simulink model "model_SCARA_PD"  (R2022b)
settings: Solver=VariableStepAuto  StartTime=0.0  StopTime=times_way(end)  RelTol=1e-3
undefined symbols (not defined in the file or in its folder): dt_animation, phi_0, psi_0, q1_0, q1_dot_0, q2_0, q2_dot_0, q3_0, q3_dot_0, q4_0, q4_dot_0, theta_0, x_0, y_0, z_0
libraries: robotcorelib x1
settings Model: Creator=anton  LastModifiedBy=angel

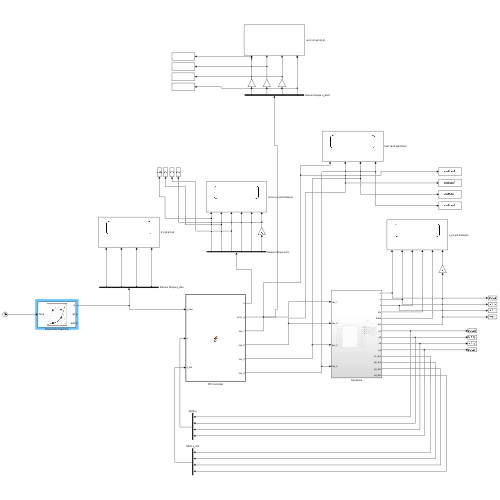
[thumbnail: Simulink's stored preview of the top-level diagram]
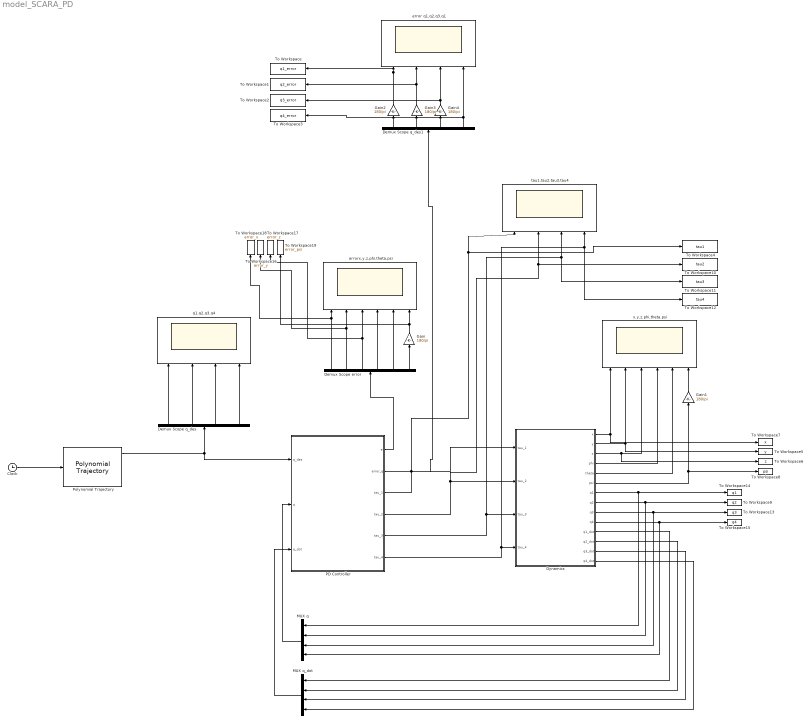
== system model_SCARA_PD ==
  Clock : Clock
  Demux Scope error : Demux  Outputs=6
  Demux Scope q_des : Demux
  Demux Scope q_des1 : Demux
  Dynamics : Subsystem
  Gain{,1..4} (5 alike) : Gain  Gain=180/pi
  MUX q : Mux
  MUX q_dot : Mux
  PD Controller : MATLAB Function  TreatAsAtomicUnit=on
  Polynomial Trajectory : robotcorelib/Polynomial Trajectory  WaypointSource=Internal  Waypoints=waypoints  TimePoints=times_way  TimeInterval=[ 1, 4 ]  Method=Cubic Polynomial  ParameterSource=Internal  VelocityBoundaryCondition=vel_boundary_condit  AccelerationBoundaryCondition=zeros( 2, 5 )  SimulateUsing=Interpreted execution
  To Workspace : ToWorkspace  VariableName=q1_error  SampleTime=dt_animation
  To Workspace1 : ToWorkspace  VariableName=q2_error  SampleTime=dt_animation
  To Workspace10 : ToWorkspace  VariableName=tau2  SampleTime=dt_animation
  To Workspace11 : ToWorkspace  VariableName=tau3  SampleTime=dt_animation
  To Workspace12 : ToWorkspace  VariableName=tau4  SampleTime=dt_animation
  To Workspace13 : ToWorkspace  VariableName=q3  SampleTime=dt_animation
  To Workspace14 : ToWorkspace  VariableName=q1  SampleTime=dt_animation
  To Workspace15 : ToWorkspace  VariableName=q4  SampleTime=dt_animation
  To Workspace16 : ToWorkspace  VariableName=error_y  SampleTime=dt_animation
  To Workspace17 : ToWorkspace  VariableName=error_z  SampleTime=dt_animation
  To Workspace18 : ToWorkspace  VariableName=error_x  SampleTime=dt_animation
  To Workspace19 : ToWorkspace  VariableName=error_psi  SampleTime=dt_animation
  To Workspace2 : ToWorkspace  VariableName=q3_error  SampleTime=dt_animation
  To Workspace3 : ToWorkspace  VariableName=q4_error  SampleTime=dt_animation
  To Workspace4 : ToWorkspace  VariableName=tau1  SampleTime=dt_animation
  To Workspace5 : ToWorkspace  VariableName=y  SampleTime=dt_animation
  To Workspace6 : ToWorkspace  VariableName=z  SampleTime=dt_animation
  To Workspace7 : ToWorkspace  VariableName=x  SampleTime=dt_animation
  To Workspace8 : ToWorkspace  VariableName=psi  SampleTime=dt_animation
  To Workspace9 : ToWorkspace  VariableName=q2  SampleTime=dt_animation
  error q1,q2,q3,q1 : Scope  NumInputPorts=4
  errorx,y,z,phi,theta,psi : Scope  NumInputPorts=6
  q1,q2,q3,q4 : Scope  NumInputPorts=4
  tau1,tau2,tau3,tau4 : Scope  NumInputPorts=4
  x,y,z,phi,theta,psi : Scope  NumInputPorts=6
  wires:
  Dynamics/7(q1) -> To Workspace14/1, MUX q/1
  Dynamics/8(q2) -> To Workspace9/1, MUX q/2
  Dynamics/9(q3) -> To Workspace13/1, MUX q/3
  Dynamics/10(q4) -> To Workspace15/1, MUX q/4
  Dynamics/11(q1_dot) -> MUX q_dot/1
  Dynamics/12(q2_dot) -> MUX q_dot/2
  Dynamics/13(q3_dot) -> MUX q_dot/3
  Dynamics/14(q4_dot) -> MUX q_dot/4
  MUX q/1 -> PD Controller/2(q)
  MUX q_dot/1 -> PD Controller/3(q_dot)
  Clock/1 -> Polynomial Trajectory/1
  Polynomial Trajectory/1 -> Demux Scope q_des/1, PD Controller/1(q_des)
  Demux Scope q_des/1 -> q1,q2,q3,q4/1
  Demux Scope q_des/2 -> q1,q2,q3,q4/2
  Demux Scope q_des/3 -> q1,q2,q3,q4/3
  Demux Scope q_des/4 -> q1,q2,q3,q4/4
  Demux Scope error/4 -> errorx,y,z,phi,theta,psi/4
  Demux Scope error/3 -> To Workspace17/1, errorx,y,z,phi,theta,psi/3
  Demux Scope error/2 -> To Workspace16/1, errorx,y,z,phi,theta,psi/2
  Demux Scope error/1 -> To Workspace18/1, errorx,y,z,phi,theta,psi/1
  Demux Scope error/5 -> errorx,y,z,phi,theta,psi/5
  Demux Scope error/6 -> Gain/1
  PD Controller/1(e) -> Demux Scope error/1
  Dynamics/6(psi) -> To Workspace8/1, Gain1/1
  Dynamics/1(x) -> To Workspace7/1, x,y,z,phi,theta,psi/1
  Dynamics/2(y) -> To Workspace5/1, x,y,z,phi,theta,psi/2
  Dynamics/3(z) -> To Workspace6/1, x,y,z,phi,theta,psi/3
  Dynamics/4(phi) -> x,y,z,phi,theta,psi/4
  Dynamics/5(theta) -> x,y,z,phi,theta,psi/5
  Gain/1 -> To Workspace19/1, errorx,y,z,phi,theta,psi/6
  PD Controller/6(tau_4) -> tau1,tau2,tau3,tau4/4, To Workspace12/1, Dynamics/4(tau_4)
  PD Controller/5(tau_3) -> tau1,tau2,tau3,tau4/3, To Workspace11/1, Dynamics/3(tau_3)
  PD Controller/4(tau_2) -> tau1,tau2,tau3,tau4/2, To Workspace10/1, Dynamics/2(tau_2)
  PD Controller/3(tau_1) -> tau1,tau2,tau3,tau4/1, To Workspace4/1, Dynamics/1(tau_1)
  Gain1/1 -> x,y,z,phi,theta,psi/6
  PD Controller/2(error_q) -> Demux Scope q_des1/1
  Demux Scope q_des1/2 -> Gain3/1
  Demux Scope q_des1/1 -> Gain2/1
  Demux Scope q_des1/3 -> Gain4/1
  Demux Scope q_des1/4 -> To Workspace3/1, error q1,q2,q3,q1/4
  Gain2/1 -> To Workspace/1, error q1,q2,q3,q1/1
  Gain3/1 -> error q1,q2,q3,q1/2, To Workspace1/1
  Gain4/1 -> error q1,q2,q3,q1/3, To Workspace2/1

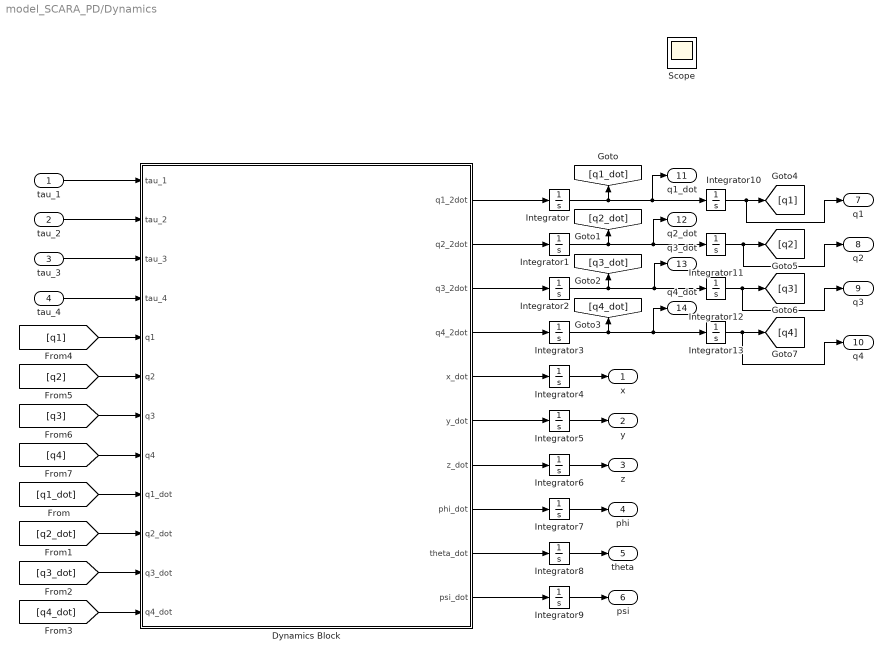
== system model_SCARA_PD/Dynamics ==
  tau_1 : Inport
  tau_2 : Inport  Port=2
  tau_3 : Inport  Port=3
  tau_4 : Inport  Port=4
  Dynamics Block : MATLAB Function  TreatAsAtomicUnit=on
  Integrator : Integrator  InitialCondition=q1_dot_0
  Integrator1 : Integrator  InitialCondition=q2_dot_0
  Integrator10 : Integrator  InitialCondition=q1_0  WrapState=on
  Integrator11 : Integrator  InitialCondition=q2_0  WrapState=on
  Integrator12 : Integrator  InitialCondition=q3_0  WrapState=on
  Integrator13 : Integrator  InitialCondition=q4_0
  Integrator2 : Integrator  InitialCondition=q3_dot_0
  Integrator3 : Integrator  InitialCondition=q4_dot_0
  Integrator4 : Integrator  InitialCondition=x_0
  Integrator5 : Integrator  InitialCondition=y_0
  Integrator6 : Integrator  InitialCondition=z_0
  Integrator7 : Integrator  InitialCondition=phi_0
  Integrator8 : Integrator  InitialCondition=theta_0
  Integrator9 : Integrator  InitialCondition=psi_0
  Scope : Scope  NumInputPorts=4
  x : Outport
  y : Outport  Port=2
  z : Outport  Port=3
  phi : Outport  Port=4
  theta : Outport  Port=5
  psi : Outport  Port=6
  q1 : Outport  Port=7
  q2 : Outport  Port=8
  q3 : Outport  Port=9
  q4 : Outport  Port=10
  q1_dot : Outport  Port=11
  q2_dot : Outport  Port=12
  q3_dot : Outport  Port=13
  q4_dot : Outport  Port=14
  wires:
  Dynamics Block/1(q1_2dot) -> Integrator/1
  Dynamics Block/2(q2_2dot) -> Integrator1/1
  Dynamics Block/3(q3_2dot) -> Integrator2/1
  Dynamics Block/4(q4_2dot) -> Integrator3/1
  Integrator/1 -> Integrator10/1, q1_dot/1, [q1_dot]
  [q1_dot] -> Dynamics Block/9(q1_dot)
  Integrator1/1 -> q2_dot/1, Integrator11/1, [q2_dot]
  Integrator2/1 -> q3_dot/1, Integrator12/1, [q3_dot]
  Integrator3/1 -> q4_dot/1, Integrator13/1, [q4_dot]
  [q2_dot] -> Dynamics Block/10(q2_dot)
  Integrator10/1 -> q1/1, [q1]
  Integrator11/1 -> q2/1, [q2]
  Integrator12/1 -> [q3], q3/1
  Integrator13/1 -> q4/1, [q4]
  [q3_dot] -> Dynamics Block/11(q3_dot)
  [q4_dot] -> Dynamics Block/12(q4_dot)
  [q1] -> Dynamics Block/5(q1)
  [q2] -> Dynamics Block/6(q2)
  [q3] -> Dynamics Block/7(q3)
  [q4] -> Dynamics Block/8(q4)
  Integrator4/1 -> x/1
  Integrator5/1 -> y/1
  Integrator6/1 -> z/1
  Integrator7/1 -> phi/1
  Integrator8/1 -> theta/1
  Integrator9/1 -> psi/1
  Dynamics Block/5(x_dot) -> Integrator4/1
  Dynamics Block/6(y_dot) -> Integrator5/1
  Dynamics Block/7(z_dot) -> Integrator6/1
  Dynamics Block/8(phi_dot) -> Integrator7/1
  Dynamics Block/9(theta_dot) -> Integrator8/1
  Dynamics Block/10(psi_dot) -> Integrator9/1
  tau_4/1 -> Dynamics Block/4(tau_4)
  tau_3/1 -> Dynamics Block/3(tau_3)
  tau_2/1 -> Dynamics Block/2(tau_2)
  tau_1/1 -> Dynamics Block/1(tau_1)

== matlab function model_SCARA_PD/PD Controller ==
  data: e output; error_q output; q_des input size=[4 1]; q input size=[4,1]; tau_1 output size=1; tau_2 output size=1; tau_3 output size=1; tau_4 output size=1; q_dot input size=[4,1]
function [e,error_q,tau_1,tau_2,tau_3,tau_4] = PD(q_des,q,q_dot)


% masses

m1 = 20; % [kg]
m2 = 15; % [kg]
m3 = 15; % [kg]
m4 = 0.5; % [kg]

% link length

l0 = 0; % [m]
l1 = 0.2; % [m]
l2 = 0.25; % [m]

% lenght joint to COM

r1 = 0.1; % [m]
r2 = 0.125; % [m]

% inertia

Iz1 = 0.27; % [kg*m^2]
Iz2 = 0.31; % [kg*m^2]
Iz3 = 0.02; % [kg*m^2]
Iz4 = 0.0001; % [kg*m^2]

g = 9.81;

G = [0; 
     0; 
     0; 
     m4*g];

q1_des = q_des(1);
q2_des = q_des(2);
q3_des = q_des(3);
q4_des = q_des(4);

q1 = q(1);
q2 = q(2);
q3 = q(3);
q4 = q(4);

eta = [- l2*sin(q1 + q2) - l1*sin(q1); 
        l2*cos(q1 + q2) + l1*cos(q1); 
        l0 + q4; 
        0; 
        0; 
        wrapToPi(q1 + q2 + q3)];

eta_des = [- l2*sin(q1_des + q2_des) - l1*sin(q1_des); 
        l2*cos(q1_des + q2_des) + l1*cos(q1_des); 
        l0 + q4_des; 
        0; 
        0; 
        wrapToPi(q1_des + q2_des + q3_des)];

e = eta_des - eta;
error_q = q_des - q;
alpha = eta_des(6) - eta(6); % errore su psi

if(alpha > 0)
    if(alpha > 2*pi - alpha)
        e(6) = - (2*pi - alpha);
    else
        e(6) = alpha;
    end

else
    alpha = -alpha;
    if(alpha > 2*pi - alpha)
        e(6) =  2*pi - alpha;
    else
        e(6) = -alpha;
    end
end

J = [- l2*cos(q1 + q2) - l1*cos(q1), -l2*cos(q1 + q2), (0), (0);
            - l2*sin(q1 + q2) - l1*sin(q1), -l2*sin(q1 + q2), (0), (0);
            (0), (0), (0), (1);
            (0), (0), (0), (0);
            (0), (0), (0), (0);
            (1), (1), (1), (0)];
    
kp1 = 1;
kp2 = 1;
kp3 = 1;
kp4 = 1;
kp5 = 1;
kp6 = 1;

kv1 = 1;
kv2 = 1;
kv3 = 1;
kv4 = 1;


Kp = 10000*diag([kp1, kp2, kp3, kp4, kp5, kp6]);
Kv = 10*diag([kv1, kv2, kv3, kv4]);

tau = J' * Kp * e - Kv * q_dot + G;
tau_1 = tau(1);
tau_2 = tau(2);
tau_3 = tau(3);
tau_4 = tau(4);

end

== matlab function model_SCARA_PD/Dynamics/Dynamics Block ==
  data: q1_2dot output size=1; q2_2dot output size=1; q3_2dot output size=1; q4_2dot output size=1; tau_1 input size=1; tau_2 input size=1; tau_3 input size=1; tau_4 input size=1; q1 input size=1; q2 input size=1; q3 input size=1; q4 input size=1; q1_dot input size=1; q2_dot input size=1; q3_dot input size=1; q4_dot input size=1; x_dot output; y_dot output; z_dot output; phi_dot output; theta_dot output; psi_dot output
function [q1_2dot, q2_2dot, q3_2dot, q4_2dot, x_dot,y_dot,z_dot,phi_dot,theta_dot,psi_dot] = Dynamics(tau_1,tau_2,tau_3,tau_4, q1,q2,q3,q4,q1_dot,q2_dot,q3_dot,q4_dot)

% Dynamic Model --> tau = M(q)*q_2dot + C(q,q_dot)*q_dot + G(q)
%
%% Parameters Definition

% masses

m1 = 20; % [kg]
m2 = 15; % [kg]
m3 = 15; % [kg]
m4 = 0.5; % [kg]

% link length

l0 = 0; % [m]
l1 = 0.2; % [m]
l2 = 0.25; % [m]
l_j1j2 = 0.02; % [m]

% lenght joint to COM

r1 = 0.1; % [m]
r2 = 0.125; % [m]

% inertia

Iz1 = 0.27; % [kg*m^2]
Iz2 = 0.31; % [kg*m^2]
Iz3 = 0.02; % [kg*m^2]
Iz4 = 0.0001; % [kg*m^2]

% gravity
g = 9.81; % [m/s^2]

%% Parameters for Matrices

alpha = Iz1 + r1^2*m1 + l1^2*m2 + l1^2*m3 + l1^2*m4;
beta = Iz2 + Iz3 + Iz4 + l2^2*m3 + l2^2*m4 + m2*r2^2;
gamma = l1*l2*m3 + l1*l2*m4 + l1*m2*r2;
delta = Iz3 + Iz4;

%% Dynamic Matrices

M = [alpha + beta + 2*gamma*cos(q2), beta + gamma*cos(q2), delta, 0;
    beta + gamma*cos(q2),                   beta,          delta, 0;
            delta,                          delta,         delta, 0; 
            0,                              0,                0, m4];

M_inv = eye(size(M))/M;

C = [-gamma*sin(q2)*q2_dot, -gamma*sin(q2)*(q1_dot + q2_dot), 0, 0;
    gamma*sin(q2) * q1_dot,             0,                    0, 0;
            0,                          0,                    0, 0; 
            0,                          0,                    0, 0];

G = [0; 0; 0; m4*g];

J = [- l2*cos(q1 + q2) - l1*cos(q1), -l2*cos(q1 + q2), (0), (0);
            - l2*sin(q1 + q2) - l1*sin(q1), -l2*sin(q1 + q2), (0), (0);
            (0), (0), (0), (1);
            (0), (0), (0), (0);
            (0), (0), (0), (0);
            (1), (1), (1), (0)];

%% Dynamics

q_dot = [q1_dot, q2_dot, q3_dot, q4_dot]';

tau = [tau_1, tau_2, tau_3, tau_4]';

% joint variable dynamics
q_2dot = M_inv*(tau - C*q_dot - G);


q1_2dot = q_2dot(1);
q2_2dot = q_2dot(2);
q3_2dot = q_2dot(3);
q4_2dot = q_2dot(4);


% End effector position dynamics
eta_dot = J*q_dot;

x_dot = eta_dot(1);
y_dot = eta_dot(2);
z_dot = eta_dot(3);
phi_dot = eta_dot(4);
theta_dot = eta_dot(5);
psi_dot = eta_dot(6);

end
